simulink model "vehicles"  (Simulink 6.5)
settings: Solver=ode45  StartTime=0.0  StopTime=50  FixedStep=.1  RelTol=1e-3
PreLoadFcn:
  | vehicledata; % load in workspace variables
  | h=frontend; % bring up GUI
  | movegui(h,'northwest') % move gui to top right
PostLoadFcn:
  | rt=sfroot; chart=rt.find('-isa', 'Stateflow.Chart', '-and', 'Name','uav_modes'); chart.view;
undefined symbols (not defined in the file or in its folder): Cd0, Clmax, Clmin, g, initthis, k, magnitude, mat2cell, num_ac, num_instincts, obstacles, omega_chi, omega_gamma, omega_v, rho, S, sigma_a, sigma_o, sigma_t1, sigma_t2, targets, Tmax, W
libraries: dspmtrx3 x38, dspindex x5, dspstat3 x4, vrlib x2
(part 2 of 2)

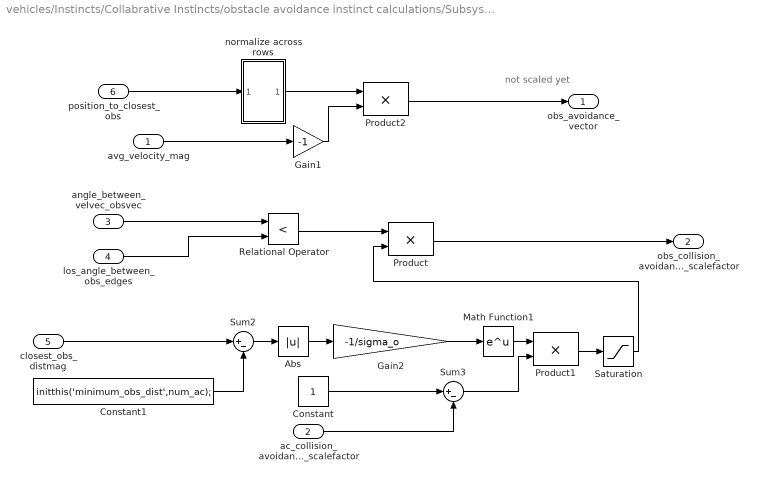
== system vehicles/Instincts/Collabrative Instincts/obstacle avoidance instinct calculations/Subsystem ==
  note: not scaled yet
  avg_velocity_mag : Inport
  ac_collision_avoidance_scalefactor : Inport  Port=2
  angle_between_velvec_obsvec : Inport  Port=3
  los_angle_between_obs_edges : Inport  Port=4
  closest_obs_distmag : Inport  Port=5
  position_to_closest_obs : Inport  Port=6
  Abs : Abs  SaturateOnIntegerOverflow=on  SampleTime=-1
  Constant : Constant  Value=1  OutDataType=sfix(16)  ConRadixGroup=Use specified scaling  OutScaling=2^0  SampleTime=inf  FramePeriod=inf
  Constant1 : Constant  Value=initthis('minimum_obs_dist',num_ac);  OutDataType=sfix(16)  ConRadixGroup=Use specified scaling  OutScaling=2^0  SampleTime=inf  FramePeriod=inf
  Gain1 : Gain  Gain=-1  SaturateOnIntegerOverflow=on
  Gain2 : Gain  Gain=-1/sigma_o  SaturateOnIntegerOverflow=on
  Math Function1 : Math  SaturateOnIntegerOverflow=on
  Product : Product  SaturateOnIntegerOverflow=on  InputSameDT=on
  Product1 : Product  SaturateOnIntegerOverflow=on  InputSameDT=on
  Product2 : Product  SaturateOnIntegerOverflow=on  InputSameDT=on
  Relational Operator : RelationalOperator  Operator=<  InputSameDT=on
  Saturation : Saturate  UpperLimit=1  LowerLimit=0
  Sum2 : Sum  Inputs=|+-  SaturateOnIntegerOverflow=on  InputSameDT=on
  Sum3 : Sum  Inputs=|+-  SaturateOnIntegerOverflow=on  InputSameDT=on
  normalize across rows : Subsystem
  obs_avoidance_vector : Outport
  obs_collision_avoidance_scalefactor : Outport  Port=2
  wires:
  angle_between_velvec_obsvec/1 -> Relational Operator/1
  los_angle_between_obs_edges/1 -> Relational Operator/2
  Relational Operator/1 -> Product/1
  closest_obs_distmag/1 -> Sum2/1
  Constant1/1 -> Sum2/2
  Sum2/1 -> Abs/1
  Gain2/1 -> Math Function1/1
  Abs/1 -> Gain2/1
  Constant/1 -> Sum3/1
  ac_collision_avoidance_scalefactor/1 -> Sum3/2
  Math Function1/1 -> Product1/1
  Sum3/1 -> Product1/2
  Product1/1 -> Saturation/1
  Saturation/1 -> Product/2
  Product/1 -> obs_collision_avoidance_scalefactor/1
  position_to_closest_obs/1 -> normalize across rows/1(In1)
  normalize across rows/1(Out1) -> Product2/1
  avg_velocity_mag/1 -> Gain1/1
  Gain1/1 -> Product2/2
  Product2/1 -> obs_avoidance_vector/1

== system vehicles/Instincts/Collabrative Instincts/target aquisition instinct calculations/desired heading and velocity capture ==
  In1 : Inport
  Abs : Abs  SaturateOnIntegerOverflow=on  SampleTime=-1
  Constant1 : Constant  Value=initthis('desired_vel',num_ac);  OutDataType=sfix(16)  ConRadixGroup=Use specified scaling  OutScaling=2^0  SampleTime=inf  FramePeriod=inf
  Constant3 : Constant  Value=1  OutDataType=sfix(16)  ConRadixGroup=Use specified scaling  OutScaling=2^0  SampleTime=inf  FramePeriod=inf
  Gain1 : Gain  Gain=-1  SaturateOnIntegerOverflow=on
  Gain2 : Gain  Gain=1/sigma_t1  SaturateOnIntegerOverflow=on
  Math Function1 : Math  Operator=sqrt  SaturateOnIntegerOverflow=on
  Math Function2 : Math  Operator=square  SaturateOnIntegerOverflow=on
  Math Function4 : Math  Operator=square  SaturateOnIntegerOverflow=on
  Math Function5 : Math  SaturateOnIntegerOverflow=on
  Matrix Sum : dspmtrx3/Matrix Sum  DialogController=dspDDGCreate  DialogControllerArgs=DataTag15  Dim=Rows  roundingMode=Floor  overflowMode=off
  Sum1 : Sum  Inputs=|+-  SaturateOnIntegerOverflow=on  InputSameDT=on
  Sum2 : Sum  Inputs=|+-  SaturateOnIntegerOverflow=on  InputSameDT=on
  "[x_dot y_dot h_dot]" : Subsystem
  velocity vectors of each AC : Concatenate  NumInputs=3  Mode=Horizontal matrix concatenation
  desired_velvec1 : Outport
  tgt_aquire_scalefactor1 : Outport  Port=2
  wires:
  "[x_dot y_dot h_dot]"/3(h_dot) -> velocity vectors of each AC/3
  "[x_dot y_dot h_dot]"/2(y_dot) -> velocity vectors of each AC/2
  "[x_dot y_dot h_dot]"/1(x_dot) -> velocity vectors of each AC/1
  velocity vectors of each AC/1 -> Sum1/2
  Sum1/1 -> Math Function2/1
  Math Function2/1 -> Matrix Sum/1
  Math Function1/1 -> [vel_error_mag]
  Matrix Sum/1 -> Math Function1/1
  [vel_error_mag] -> Gain2/1
  Gain2/1 -> Math Function4/1
  Math Function4/1 -> Gain1/1
  Math Function5/1 -> Sum2/1
  Constant3/1 -> Sum2/2
  Sum2/1 -> Abs/1
  In1/1 -> "[x_dot y_dot h_dot]"/1(States)
  Abs/1 -> tgt_aquire_scalefactor1/1
  Gain1/1 -> Math Function5/1
  Constant1/1 -> Sum1/1, desired_velvec1/1

== system vehicles/Instincts/Collabrative Instincts/target aquisition instinct calculations/target capture ==
  In1 : Inport
  In2 : Inport  Port=2
  tgt_aquire_on : Inport  Port=3
  If : If
  If Action Subsystem : Subsystem  TreatAsAtomicUnit=on
  If Action Subsystem1 : Subsystem  TreatAsAtomicUnit=on
  Merge : Merge
  Merge1 : Merge
  Transpose : dspmtrx3/Transpose  SystemSampleTime=-1  Hermitian=off  overflowFlag=on
  tgt_aquire_scalefactor2 : Outport
  desired_velvec2 : Outport  Port=2
  wires:
  tgt_aquire_on/1 -> If/1
  If/1 -> If Action Subsystem/Action
  If/2 -> If Action Subsystem1/Action
  If Action Subsystem/1(tgt_aquire_scalefactor2) -> Merge/1
  If Action Subsystem1/1(tgt_aquire_scalefactor2) -> Merge/2
  If Action Subsystem1/2(desired_velvec2) -> Merge1/2
  If Action Subsystem/2(desired_velvec2) -> Merge1/1
  Merge/1 -> Transpose/1
  In1/1 -> If Action Subsystem/1(States)
  In2/1 -> If Action Subsystem/2(avg_velocity_mag)
  Transpose/1 -> tgt_aquire_scalefactor2/1
  Merge1/1 -> desired_velvec2/1

== system vehicles/Vehicle/EOM/[Velocity_dot gamma_dot chi_dot]/Subsystem ==
  Velocity : Inport
  loadfactor : Inport  Port=2
  Gain1 : Gain  Gain=.5*rho*S*Cd0  SaturateOnIntegerOverflow=on
  Gain2 : Gain  Gain=2*k*W^2/(rho*S)  SaturateOnIntegerOverflow=on
  Math Function : Math  Operator=square  SaturateOnIntegerOverflow=on
  Math Function1 : Math  Operator=square  SaturateOnIntegerOverflow=on
  Product : Product  Inputs=/*  SaturateOnIntegerOverflow=on  InputSameDT=on
  Sum : Sum  Inputs=|++  SaturateOnIntegerOverflow=on  InputSameDT=on
  Drag : Outport
  wires:
  Velocity/1 -> Math Function/1
  Math Function/1 -> Gain1/1, Product/1
  loadfactor/1 -> Math Function1/1
  Math Function1/1 -> Product/2
  Product/1 -> Gain2/1
  Gain2/1 -> Sum/2
  Gain1/1 -> Sum/1
  Sum/1 -> Drag/1

== system vehicles/Instincts/Collabrative Instincts/AC avoidance instinct calculations/Distance between AC Calculator1/For Iterator Subsystem ==
  num_ac : Inport
  positions : Inport  Port=2
  position : Inport  Port=3
  initial row : Inport  Port=4
  row : Inport  Port=5
  Assignment : Assignment  InputType=Matrix  IndexIsStartValue=off  ElementSrc=External  Elements=1  RowSrc=Internal  Rows=1  ColumnSrc=External  Columns=1  OutputDimensions=[1 1]
  Constant : Constant  Value=1e099  OutDataType=sfix(16)  ConRadixGroup=Use specified scaling  OutScaling=2^0  SampleTime=inf  FramePeriod=inf
  For Iterator : ForIterator  IterationSource=external  IterationVariableDataType=double
  Math Function : Math  Operator=magnitude^2  SaturateOnIntegerOverflow=on
  Math Function1 : Math  Operator=sqrt  SaturateOnIntegerOverflow=on
  Matrix Sum : dspmtrx3/Matrix Sum  DialogController=dspDDGCreate  DialogControllerArgs=DataTag1  Dim=Rows  roundingMode=Floor  overflowMode=off
  Relational Operator : RelationalOperator  Operator===  InputSameDT=on
  Selector : Selector  InputType=Matrix  ElementSrc=Internal  Elements=[1 3]  RowSrc=External  Rows=1  ColumnSrc=Internal  Columns=-1  InputPortWidth=3  IndexIsStartValue=off
  Sum : Sum  Inputs=|-+  SaturateOnIntegerOverflow=on  InputSameDT=on
  Switch1 : Switch  Threshold=.5  SaturateOnIntegerOverflow=on  InputSameDT=on
  row for one aircraft : Outport
  wires:
  num_ac/1 -> For Iterator/1
  For Iterator/1 -> Selector/2, Relational Operator/1, Assignment/3
  positions/1 -> Selector/1
  position/1 -> Sum/1
  Selector/1 -> Sum/2
  Sum/1 -> Math Function/1
  Math Function/1 -> Matrix Sum/1
  Matrix Sum/1 -> Math Function1/1
  Relational Operator/1 -> Switch1/2
  Switch1/1 -> Assignment/2
  Math Function1/1 -> Switch1/3
  Constant/1 -> Switch1/1
  row/1 -> Relational Operator/2
  initial row/1 -> Assignment/1
  Assignment/1 -> row for one aircraft/1

== system vehicles/Instincts/Collabrative Instincts/obstacle avoidance instinct calculations/Angle calulator/[x_dot y_dot h_dot] ==
  States : Inport
  Product : Product  Inputs=3  SaturateOnIntegerOverflow=on  InputSameDT=on
  Product1 : Product  SaturateOnIntegerOverflow=on  InputSameDT=on
  Product2 : Product  Inputs=3  SaturateOnIntegerOverflow=on  InputSameDT=on
  "V, gamma, chi" : BusSelector  OutputSignals=Velocity,gamma,chi
  cos_chi : Trigonometry  Operator=cos
  cos_gamma : Trigonometry  Operator=cos
  sin_chi : Trigonometry
  sin_gamma : Trigonometry
  x_dot : Outport
  y_dot : Outport  Port=2
  h_dot : Outport  Port=3
  wires:
  "V, gamma, chi"/1 -> Product2/1, Product/1, Product1/1  "<Velocity>"
  "V, gamma, chi"/2 -> sin_gamma/1, cos_gamma/1  "<gamma>"
  "V, gamma, chi"/3 -> sin_chi/1, cos_chi/1  "<chi>"
  cos_gamma/1 -> Product2/2, Product/2
  cos_chi/1 -> Product2/3
  sin_chi/1 -> Product/3
  sin_gamma/1 -> Product1/2
  States/1 -> "V, gamma, chi"/1
  Product2/1 -> x_dot/1  "x_dot"
  Product/1 -> y_dot/1  "y_dot"
  Product1/1 -> h_dot/1  "h_dot"

== system vehicles/Instincts/Collabrative Instincts/obstacle avoidance instinct calculations/Angle calulator/normalize across rows ==
  In1 : Inport
  Math Function : Math  Operator=square  SaturateOnIntegerOverflow=on
  Math Function1 : Math  Operator=sqrt  SaturateOnIntegerOverflow=on
  Math Function2 : Math  Operator=reciprocal  SaturateOnIntegerOverflow=on
  Matrix Scaling : dspmtrx3/Matrix Scaling  DialogController=dspDDGCreate  DialogControllerArgs=DataTag7  mode=Scale rows (D*A)  D_Source=Input port  D_VectFromMask=[0.5 0.25]  roundingMode=Floor  overflowMode=off
  Matrix Sum : dspmtrx3/Matrix Sum  DialogController=dspDDGCreate  DialogControllerArgs=DataTag8  Dim=Rows  roundingMode=Floor  overflowMode=off
  Out1 : Outport
  wires:
  In1/1 -> Matrix Scaling/1, Math Function/1
  Math Function/1 -> Matrix Sum/1
  Matrix Sum/1 -> Math Function1/1
  Math Function1/1 -> Math Function2/1
  Math Function2/1 -> Matrix Scaling/2
  Matrix Scaling/1 -> Out1/1

== system vehicles/Instincts/Collabrative Instincts/obstacle avoidance instinct calculations/Angle calulator/normalize across rows1 ==
  In1 : Inport
  Math Function : Math  Operator=square  SaturateOnIntegerOverflow=on
  Math Function1 : Math  Operator=sqrt  SaturateOnIntegerOverflow=on
  Math Function2 : Math  Operator=reciprocal  SaturateOnIntegerOverflow=on
  Matrix Scaling : dspmtrx3/Matrix Scaling  DialogController=dspDDGCreate  DialogControllerArgs=DataTag9  mode=Scale rows (D*A)  D_Source=Input port  D_VectFromMask=[0.5 0.25]  roundingMode=Floor  overflowMode=off
  Matrix Sum : dspmtrx3/Matrix Sum  DialogController=dspDDGCreate  DialogControllerArgs=DataTag10  Dim=Rows  roundingMode=Floor  overflowMode=off
  Out1 : Outport
  wires:
  In1/1 -> Matrix Scaling/1, Math Function/1
  Math Function/1 -> Matrix Sum/1
  Matrix Sum/1 -> Math Function1/1
  Math Function1/1 -> Math Function2/1
  Math Function2/1 -> Matrix Scaling/2
  Matrix Scaling/1 -> Out1/1

== system vehicles/Instincts/Collabrative Instincts/obstacle avoidance instinct calculations/Distance from obstacles Calculator/For Iterator Subsystem ==
  note: filling in columns at a time.
      | ie distance to each obstacle from
      | a given aircraft.
      | [num_obs, num_ac]
  position of obs : Inport
  num_obs : Inport  Port=2
  position of ac : Inport  Port=3
  initial column : Inport  Port=4
  Assignment : Assignment  InputType=Vector  IndexIsStartValue=off  ElementSrc=External  Elements=1  RowSrc=External  Rows=1  ColumnSrc=External  Columns=1  OutputDimensions=[1 1]
  For Iterator : ForIterator  IterationSource=external  IterationVariableDataType=double
  Math Function : Math  Operator=magnitude^2  SaturateOnIntegerOverflow=on
  Math Function1 : Math  Operator=sqrt  SaturateOnIntegerOverflow=on
  Matrix Sum : dspmtrx3/Matrix Sum  DialogController=dspDDGCreate  DialogControllerArgs=DataTag11  Dim=Rows  roundingMode=Floor  overflowMode=off
  Selector : Selector  InputType=Matrix  ElementSrc=Internal  Elements=[1 3]  RowSrc=External  Rows=1  ColumnSrc=Internal  Columns=-1  InputPortWidth=3  IndexIsStartValue=off
  Sum : Sum  Inputs=|-+  SaturateOnIntegerOverflow=on  InputSameDT=on
  row for one obstacle : Outport
  wires:
  num_obs/1 -> For Iterator/1
  For Iterator/1 -> Selector/2, Assignment/3
  position of obs/1 -> Selector/1
  position of ac/1 -> Sum/1
  Selector/1 -> Sum/2
  Sum/1 -> Math Function/1
  Math Function/1 -> Matrix Sum/1
  Matrix Sum/1 -> Math Function1/1
  Math Function1/1 -> Assignment/2
  initial column/1 -> Assignment/1
  Assignment/1 -> row for one obstacle/1

== system vehicles/Instincts/Collabrative Instincts/obstacle avoidance instinct calculations/Subsystem/normalize across rows ==
  In1 : Inport
  Math Function : Math  Operator=square  SaturateOnIntegerOverflow=on
  Math Function1 : Math  Operator=sqrt  SaturateOnIntegerOverflow=on
  Math Function2 : Math  Operator=reciprocal  SaturateOnIntegerOverflow=on
  Matrix Scaling : dspmtrx3/Matrix Scaling  DialogController=dspDDGCreate  DialogControllerArgs=DataTag13  mode=Scale rows (D*A)  D_Source=Input port  D_VectFromMask=[0.5 0.25]  roundingMode=Floor  overflowMode=off
  Matrix Sum : dspmtrx3/Matrix Sum  DialogController=dspDDGCreate  DialogControllerArgs=DataTag14  Dim=Rows  roundingMode=Floor  overflowMode=off
  Out1 : Outport
  wires:
  In1/1 -> Matrix Scaling/1, Math Function/1
  Math Function/1 -> Matrix Sum/1
  Matrix Sum/1 -> Math Function1/1
  Math Function1/1 -> Math Function2/1
  Math Function2/1 -> Matrix Scaling/2
  Matrix Scaling/1 -> Out1/1

== system vehicles/Instincts/Collabrative Instincts/target aquisition instinct calculations/desired heading and velocity capture/[x_dot y_dot h_dot] ==
  States : Inport
  Product : Product  Inputs=3  SaturateOnIntegerOverflow=on  InputSameDT=on
  Product1 : Product  SaturateOnIntegerOverflow=on  InputSameDT=on
  Product2 : Product  Inputs=3  SaturateOnIntegerOverflow=on  InputSameDT=on
  "V, gamma, chi" : BusSelector  OutputSignals=Velocity,gamma,chi
  cos_chi : Trigonometry  Operator=cos
  cos_gamma : Trigonometry  Operator=cos
  sin_chi : Trigonometry
  sin_gamma : Trigonometry
  x_dot : Outport
  y_dot : Outport  Port=2
  h_dot : Outport  Port=3
  wires:
  "V, gamma, chi"/1 -> Product2/1, Product/1, Product1/1  "<Velocity>"
  "V, gamma, chi"/2 -> sin_gamma/1, cos_gamma/1  "<gamma>"
  "V, gamma, chi"/3 -> sin_chi/1, cos_chi/1  "<chi>"
  cos_gamma/1 -> Product2/2, Product/2
  cos_chi/1 -> Product2/3
  sin_chi/1 -> Product/3
  sin_gamma/1 -> Product1/2
  States/1 -> "V, gamma, chi"/1
  Product2/1 -> x_dot/1  "x_dot"
  Product/1 -> y_dot/1  "y_dot"
  Product1/1 -> h_dot/1  "h_dot"

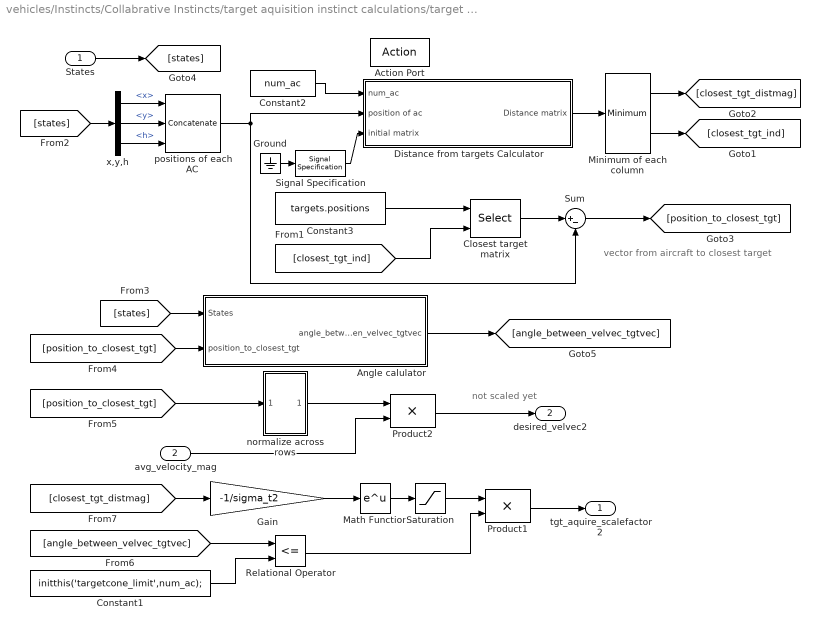
== system vehicles/Instincts/Collabrative Instincts/target aquisition instinct calculations/target capture/If Action Subsystem ==
  note: vector from aircraft to closest target
  note: not scaled yet
  States : Inport
  avg_velocity_mag : Inport  Port=2
  Action Port : ActionPort  ActionType=then
  Angle calulator : Subsystem
  Closest target matrix : Selector  InputType=Matrix  ElementSrc=Internal  Elements=[1 3]  RowSrc=External  Rows=1  ColumnSrc=Internal  Columns=-1  InputPortWidth=3  IndexIsStartValue=off
  Constant1 : Constant  Value=initthis('targetcone_limit',num_ac);  OutDataType=sfix(16)  ConRadixGroup=Use specified scaling  OutScaling=2^0  SampleTime=inf  FramePeriod=inf
  Constant2 : Constant  Value=num_ac  OutDataType=sfix(16)  ConRadixGroup=Use specified scaling  OutScaling=2^0  SampleTime=inf  FramePeriod=inf
  Constant3 : Constant  Value=targets.positions  OutDataType=sfix(16)  ConRadixGroup=Use specified scaling  OutScaling=2^0  SampleTime=inf  FramePeriod=inf
  Distance from targets Calculator : Subsystem  TreatAsAtomicUnit=on
  Gain : Gain  Gain=-1/sigma_t2  SaturateOnIntegerOverflow=on
  Ground : Ground
  Math Function : Math  SaturateOnIntegerOverflow=on
  Minimum of each column : dspstat3/Minimum  DialogController=dspfixptddg.MinMax  DialogControllerArgs=DataTag21  fcn=Value and Index  reset=None  indexBase=One  operateOver=Each column  colComp=on  operation=minimum  roundingMode=Floor  overflowMode=off
  Product1 : Product  SaturateOnIntegerOverflow=on  InputSameDT=on
  Product2 : Product  SaturateOnIntegerOverflow=on  InputSameDT=on
  Relational Operator : RelationalOperator  Operator=<=  InputSameDT=on
  Saturation : Saturate  UpperLimit=1  LowerLimit=0
  Signal Specification : SignalSpecification  Dimensions=[size(targets.positions,1),num_ac]
  Sum : Sum  Inputs=|+-  SaturateOnIntegerOverflow=on  InputSameDT=on
  normalize across rows : Subsystem
  positions of each AC : Concatenate  NumInputs=3  Mode=Horizontal matrix concatenation
  x,y,h : BusSelector  OutputSignals=x,y,h
  tgt_aquire_scalefactor2 : Outport
  desired_velvec2 : Outport  Port=2
  wires:
  Minimum of each column/1 -> [closest_tgt_distmag]
  Sum/1 -> [position_to_closest_tgt]
  Minimum of each column/2 -> [closest_tgt_ind]
  Distance from targets Calculator/1(Distance matrix) -> Minimum of each column/1
  positions of each AC/1 -> Sum/2, Distance from targets Calculator/2(position of ac)
  x,y,h/3 -> positions of each AC/3  "<h>"
  x,y,h/2 -> positions of each AC/2  "<y>"
  x,y,h/1 -> positions of each AC/1  "<x>"
  [closest_tgt_ind] -> Closest target matrix/2
  Constant3/1 -> Closest target matrix/1
  Closest target matrix/1 -> Sum/1
  States/1 -> [states]
  [states] -> x,y,h/1
  [states] -> Angle calulator/1(States)
  [position_to_closest_tgt] -> Angle calulator/2(position_to_closest_tgt)
  Angle calulator/1(angle_between_velvec_tgtvec) -> [angle_between_velvec_tgtvec]
  [position_to_closest_tgt] -> normalize across rows/1(In1)
  normalize across rows/1(Out1) -> Product2/1
  avg_velocity_mag/1 -> Product2/2
  Product2/1 -> desired_velvec2/1
  [angle_between_velvec_tgtvec] -> Relational Operator/1
  Constant1/1 -> Relational Operator/2
  Relational Operator/1 -> Product1/2
  Math Function/1 -> Saturation/1
  [closest_tgt_distmag] -> Gain/1
  Gain/1 -> Math Function/1
  Saturation/1 -> Product1/1
  Product1/1 -> tgt_aquire_scalefactor2/1
  Ground/1 -> Signal Specification/1
  Constant2/1 -> Distance from targets Calculator/1(num_ac)
  Signal Specification/1 -> Distance from targets Calculator/3(initial matrix)

== system vehicles/Instincts/Collabrative Instincts/target aquisition instinct calculations/target capture/If Action Subsystem1 ==
  Action Port : ActionPort  ActionType=else
  Ground : Ground
  Ground1 : Ground
  Signal Specification : SignalSpecification  Dimensions=[num_ac]
  Signal Specification1 : SignalSpecification  Dimensions=[num_ac,3]
  tgt_aquire_scalefactor2 : Outport
  desired_velvec2 : Outport  Port=2
  wires:
  Ground/1 -> Signal Specification/1
  Signal Specification/1 -> tgt_aquire_scalefactor2/1
  Signal Specification1/1 -> desired_velvec2/1
  Ground1/1 -> Signal Specification1/1

== system vehicles/Instincts/Collabrative Instincts/target aquisition instinct calculations/target capture/If Action Subsystem/Angle calulator ==
  States : Inport
  position_to_closest_tgt : Inport  Port=2
  Extract Diagonal : dspmtrx3/Extract Diagonal
  Matrix Multiply : Product  Multiplication=Matrix(*)
  Transpose1 : dspmtrx3/Transpose  SystemSampleTime=-1  Hermitian=off  overflowFlag=on
  Trigonometric Function : Trigonometry  Operator=acos
  "[x_dot y_dot h_dot]" : Subsystem
  normalize across rows : Subsystem
  normalize across rows1 : Subsystem
  velocity vectors of each AC : Concatenate  NumInputs=3  Mode=Horizontal matrix concatenation
  angle_between_velvec_tgtvec : Outport
  wires:
  "[x_dot y_dot h_dot]"/3(h_dot) -> velocity vectors of each AC/3
  "[x_dot y_dot h_dot]"/2(y_dot) -> velocity vectors of each AC/2
  "[x_dot y_dot h_dot]"/1(x_dot) -> velocity vectors of each AC/1
  velocity vectors of each AC/1 -> normalize across rows/1(In1)
  normalize across rows/1(Out1) -> Matrix Multiply/1
  normalize across rows1/1(Out1) -> Transpose1/1
  Transpose1/1 -> Matrix Multiply/2
  Matrix Multiply/1 -> Extract Diagonal/1
  Extract Diagonal/1 -> Trigonometric Function/1
  States/1 -> "[x_dot y_dot h_dot]"/1(States)
  Trigonometric Function/1 -> angle_between_velvec_tgtvec/1
  position_to_closest_tgt/1 -> normalize across rows1/1(In1)

== system vehicles/Instincts/Collabrative Instincts/target aquisition instinct calculations/target capture/If Action Subsystem/Distance from targets Calculator ==
  num_ac : Inport
  position of ac : Inport  Port=2
  initial matrix : Inport  Port=3
  Assignment : Assignment  InputType=Matrix  IndexIsStartValue=off  ElementSrc=External  Elements=1  RowSrc=External  Rows=1  ColumnSrc=External  Columns=1  OutputDimensions=[1 1]
  Constant : Constant  Value=[1:size(targets.positions,1)]  OutDataType=sfix(16)  ConRadixGroup=Use specified scaling  OutScaling=2^0  SampleTime=inf  FramePeriod=inf
  Constant1 : Constant  Value=targets.positions  OutDataType=sfix(16)  ConRadixGroup=Use specified scaling  OutScaling=2^0  SampleTime=inf  FramePeriod=inf
  Constant2 : Constant  Value=size(targets.positions,1)  OutDataType=sfix(16)  ConRadixGroup=Use specified scaling  OutScaling=2^0  SampleTime=inf  FramePeriod=inf
  For Iterator : ForIterator  IterationSource=external  IterationVariableDataType=double
  For Iterator Subsystem : Subsystem  TreatAsAtomicUnit=on
  Ground : Ground
  Selector : Selector  InputType=Matrix  ElementSrc=Internal  Elements=[1 3]  RowSrc=External  Rows=1  ColumnSrc=Internal  Columns=-1  InputPortWidth=3  IndexIsStartValue=off
  Signal Specification : SignalSpecification  Dimensions=[size(targets.positions,1),1]
  Distance matrix : Outport
  wires:
  num_ac/1 -> For Iterator/1
  For Iterator/1 -> Selector/2, Assignment/4
  position of ac/1 -> Selector/1
  Selector/1 -> For Iterator Subsystem/3(position of ac)
  For Iterator Subsystem/1(column for one target) -> Assignment/2
  Ground/1 -> Signal Specification/1
  Signal Specification/1 -> For Iterator Subsystem/4(initial column)
  initial matrix/1 -> Assignment/1
  Assignment/1 -> Distance matrix/1
  Constant1/1 -> For Iterator Subsystem/1(position of tgt)
  Constant/1 -> Assignment/3
  Constant2/1 -> For Iterator Subsystem/2(num_tgt)

== system vehicles/Instincts/Collabrative Instincts/target aquisition instinct calculations/target capture/If Action Subsystem/normalize across rows ==
  In1 : Inport
  Math Function : Math  Operator=square  SaturateOnIntegerOverflow=on
  Math Function1 : Math  Operator=sqrt  SaturateOnIntegerOverflow=on
  Math Function2 : Math  Operator=reciprocal  SaturateOnIntegerOverflow=on
  Matrix Scaling : dspmtrx3/Matrix Scaling  DialogController=dspDDGCreate  DialogControllerArgs=DataTag22  mode=Scale rows (D*A)  D_Source=Input port  D_VectFromMask=[0.5 0.25]  roundingMode=Floor  overflowMode=off
  Matrix Sum : dspmtrx3/Matrix Sum  DialogController=dspDDGCreate  DialogControllerArgs=DataTag23  Dim=Rows  roundingMode=Floor  overflowMode=off
  Out1 : Outport
  wires:
  In1/1 -> Matrix Scaling/1, Math Function/1
  Math Function/1 -> Matrix Sum/1
  Matrix Sum/1 -> Math Function1/1
  Math Function1/1 -> Math Function2/1
  Math Function2/1 -> Matrix Scaling/2
  Matrix Scaling/1 -> Out1/1

== system vehicles/Instincts/Collabrative Instincts/target aquisition instinct calculations/target capture/If Action Subsystem/Angle calulator/[x_dot y_dot h_dot] ==
  States : Inport
  Product : Product  Inputs=3  SaturateOnIntegerOverflow=on  InputSameDT=on
  Product1 : Product  SaturateOnIntegerOverflow=on  InputSameDT=on
  Product2 : Product  Inputs=3  SaturateOnIntegerOverflow=on  InputSameDT=on
  "V, gamma, chi" : BusSelector  OutputSignals=Velocity,gamma,chi
  cos_chi : Trigonometry  Operator=cos
  cos_gamma : Trigonometry  Operator=cos
  sin_chi : Trigonometry
  sin_gamma : Trigonometry
  x_dot : Outport
  y_dot : Outport  Port=2
  h_dot : Outport  Port=3
  wires:
  "V, gamma, chi"/1 -> Product2/1, Product/1, Product1/1  "<Velocity>"
  "V, gamma, chi"/2 -> sin_gamma/1, cos_gamma/1  "<gamma>"
  "V, gamma, chi"/3 -> sin_chi/1, cos_chi/1  "<chi>"
  cos_gamma/1 -> Product2/2, Product/2
  cos_chi/1 -> Product2/3
  sin_chi/1 -> Product/3
  sin_gamma/1 -> Product1/2
  States/1 -> "V, gamma, chi"/1
  Product2/1 -> x_dot/1  "x_dot"
  Product/1 -> y_dot/1  "y_dot"
  Product1/1 -> h_dot/1  "h_dot"

== system vehicles/Instincts/Collabrative Instincts/target aquisition instinct calculations/target capture/If Action Subsystem/Angle calulator/normalize across rows ==
  In1 : Inport
  Math Function : Math  Operator=square  SaturateOnIntegerOverflow=on
  Math Function1 : Math  Operator=sqrt  SaturateOnIntegerOverflow=on
  Math Function2 : Math  Operator=reciprocal  SaturateOnIntegerOverflow=on
  Matrix Scaling : dspmtrx3/Matrix Scaling  DialogController=dspDDGCreate  DialogControllerArgs=DataTag16  mode=Scale rows (D*A)  D_Source=Input port  D_VectFromMask=[0.5 0.25]  roundingMode=Floor  overflowMode=off
  Matrix Sum : dspmtrx3/Matrix Sum  DialogController=dspDDGCreate  DialogControllerArgs=DataTag17  Dim=Rows  roundingMode=Floor  overflowMode=off
  Out1 : Outport
  wires:
  In1/1 -> Matrix Scaling/1, Math Function/1
  Math Function/1 -> Matrix Sum/1
  Matrix Sum/1 -> Math Function1/1
  Math Function1/1 -> Math Function2/1
  Math Function2/1 -> Matrix Scaling/2
  Matrix Scaling/1 -> Out1/1

== system vehicles/Instincts/Collabrative Instincts/target aquisition instinct calculations/target capture/If Action Subsystem/Angle calulator/normalize across rows1 ==
  In1 : Inport
  Math Function : Math  Operator=square  SaturateOnIntegerOverflow=on
  Math Function1 : Math  Operator=sqrt  SaturateOnIntegerOverflow=on
  Math Function2 : Math  Operator=reciprocal  SaturateOnIntegerOverflow=on
  Matrix Scaling : dspmtrx3/Matrix Scaling  DialogController=dspDDGCreate  DialogControllerArgs=DataTag18  mode=Scale rows (D*A)  D_Source=Input port  D_VectFromMask=[0.5 0.25]  roundingMode=Floor  overflowMode=off
  Matrix Sum : dspmtrx3/Matrix Sum  DialogController=dspDDGCreate  DialogControllerArgs=DataTag19  Dim=Rows  roundingMode=Floor  overflowMode=off
  Out1 : Outport
  wires:
  In1/1 -> Matrix Scaling/1, Math Function/1
  Math Function/1 -> Matrix Sum/1
  Matrix Sum/1 -> Math Function1/1
  Math Function1/1 -> Math Function2/1
  Math Function2/1 -> Matrix Scaling/2
  Matrix Scaling/1 -> Out1/1

== system vehicles/Instincts/Collabrative Instincts/target aquisition instinct calculations/target capture/If Action Subsystem/Distance from targets Calculator/For Iterator Subsystem ==
  note: filling in columns at a time.
      | ie distance to each target from
      | a given aircraft.
      | [num_tgt, num_ac]
  position of tgt : Inport
  num_tgt : Inport  Port=2
  position of ac : Inport  Port=3
  initial column : Inport  Port=4
  Assignment : Assignment  InputType=Vector  IndexIsStartValue=off  ElementSrc=External  Elements=1  RowSrc=External  Rows=1  ColumnSrc=External  Columns=1  OutputDimensions=[1 1]
  For Iterator : ForIterator  IterationSource=external  IterationVariableDataType=double
  Math Function : Math  Operator=magnitude^2  SaturateOnIntegerOverflow=on
  Math Function1 : Math  Operator=sqrt  SaturateOnIntegerOverflow=on
  Matrix Sum : dspmtrx3/Matrix Sum  DialogController=dspDDGCreate  DialogControllerArgs=DataTag20  Dim=Rows  roundingMode=Floor  overflowMode=off
  Selector : Selector  InputType=Matrix  ElementSrc=Internal  Elements=[1 3]  RowSrc=External  Rows=1  ColumnSrc=Internal  Columns=-1  InputPortWidth=3  IndexIsStartValue=off
  Sum : Sum  Inputs=|-+  SaturateOnIntegerOverflow=on  InputSameDT=on
  column for one target : Outport
  wires:
  num_tgt/1 -> For Iterator/1
  For Iterator/1 -> Selector/2, Assignment/3
  position of tgt/1 -> Selector/1
  position of ac/1 -> Sum/1
  Selector/1 -> Sum/2
  Sum/1 -> Math Function/1
  Math Function/1 -> Matrix Sum/1
  Matrix Sum/1 -> Math Function1/1
  Math Function1/1 -> Assignment/2
  initial column/1 -> Assignment/1
  Assignment/1 -> column for one target/1

== stateflow chart Mode Display/uav_modes ==
  state uav1 [parallel]
    settings: executionOrder=1
    state ac_avoid
      en:mode_count[1][1]++;
    state obs_avoid
      en:mode_count[1][2]++;
    state tgt_aquire
      en:mode_count[1][3]++;
    state form_keep
      en:mode_count[1][4]++;
    uav1 -> uav1.ac_avoid [order 1] : aa
    uav1 -> uav1.obs_avoid [order 2] : oa
    uav1 -> uav1.form_keep [order 4] : fk
    uav1 -> uav1.tgt_aquire [order 3] : ta
    (default) -> uav1.ac_avoid
  state uav2 [parallel]
    settings: executionOrder=2
    state ac_avoid
      en:mode_count[2][1]++;
    state obs_avoid
      en:mode_count[2][2]++;
    state tgt_aquire
      en:mode_count[2][3]++;
    state form_keep
      en:mode_count[2][4]++;
    uav2 -> uav2.ac_avoid [order 1] : aa
    uav2 -> uav2.obs_avoid [order 2] : oa
    uav2 -> uav2.form_keep [order 4] : fk
    uav2 -> uav2.tgt_aquire [order 3] : ta
    (default) -> uav2.ac_avoid
  state uav3 [parallel]
    settings: executionOrder=3
    state ac_avoid
      en:mode_count[3][1]++;
    state obs_avoid
      en:mode_count[3][2]++;
    state tgt_aquire
      en:mode_count[3][3]++;
    state form_keep
      en:mode_count[3][4]++;
    uav3 -> uav3.ac_avoid [order 1] : aa
    uav3 -> uav3.obs_avoid [order 2] : oa
    uav3 -> uav3.form_keep [order 4] : fk
    uav3 -> uav3.tgt_aquire [order 3] : ta
    (default) -> uav3.ac_avoid
  state uav4 [parallel]
    settings: executionOrder=4
    state ac_avoid
      en:mode_count[4][1]++;
    state obs_avoid
      en:mode_count[4][2]++;
    state tgt_aquire
      en:mode_count[4][3]++;
    state form_keep
      en:mode_count[4][4]++;
    uav4 -> uav4.ac_avoid [order 1] : aa
    uav4 -> uav4.obs_avoid [order 2] : oa
    uav4 -> uav4.form_keep [order 4] : fk
    uav4 -> uav4.tgt_aquire [order 3] : ta
    (default) -> uav4.ac_avoid
  state uav5 [parallel]
    settings: executionOrder=5
    state ac_avoid
      en:mode_count[5][1]++;
    state obs_avoid
      en:mode_count[5][2]++;
    state tgt_aquire
      en:mode_count[5][3]++;
    state form_keep
      en:mode_count[5][4]++;
    uav5 -> uav5.ac_avoid [order 1] : aa
    uav5 -> uav5.obs_avoid [order 2] : oa
    uav5 -> uav5.form_keep [order 4] : fk
    uav5 -> uav5.tgt_aquire [order 3] : ta
    (default) -> uav5.ac_avoid
  state parse_events [parallel]
    on e1: uav1.aa;
    on e2: uav1.oa;
    on e3: uav1.ta;
    on e4: uav1.fk;
    on e5: uav2.aa;
    on e6: uav2.oa;
    on e7: uav2.ta;
    on e8: uav2.fk;
    on e9: uav3.aa;
    on e10: uav3.oa;
    on e11: uav3.ta;
    on e12: uav3.fk;
    on e13: uav4.aa;
    on e14: uav4.oa;
    on e15: uav4.ta;
    on e16: uav4.fk;
    on e17: uav5.aa;
    on e18: uav5.oa;
    on e19: uav5.ta;
    on e20: uav5.fk;
    settings: executionOrder=6
  data: mode_count local double size=[5 4]
  events: aa local EITHER_EDGE_EVENT; fk local EITHER_EDGE_EVENT; oa local EITHER_EDGE_EVENT; ta local EITHER_EDGE_EVENT; aa local EITHER_EDGE_EVENT; fk local EITHER_EDGE_EVENT; oa local EITHER_EDGE_EVENT; ta local EITHER_EDGE_EVENT; aa local EITHER_EDGE_EVENT; fk local EITHER_EDGE_EVENT; oa local EITHER_EDGE_EVENT; ta local EITHER_EDGE_EVENT; aa local EITHER_EDGE_EVENT; fk local EITHER_EDGE_EVENT; oa local EITHER_EDGE_EVENT; ta local EITHER_EDGE_EVENT; aa local EITHER_EDGE_EVENT; fk local EITHER_EDGE_EVENT; oa local EITHER_EDGE_EVENT; ta local EITHER_EDGE_EVENT; e1 input RISING_EDGE_EVENT; e2 input RISING_EDGE_EVENT; e3 input RISING_EDGE_EVENT; e4 input RISING_EDGE_EVENT; e5 input RISING_EDGE_EVENT; e6 input RISING_EDGE_EVENT; e7 input RISING_EDGE_EVENT; e8 input RISING_EDGE_EVENT; e9 input RISING_EDGE_EVENT; e10 input RISING_EDGE_EVENT; e11 input RISING_EDGE_EVENT; e12 input RISING_EDGE_EVENT; e13 input RISING_EDGE_EVENT; e14 input RISING_EDGE_EVENT; e15 input RISING_EDGE_EVENT; e16 input RISING_EDGE_EVENT; e17 input RISING_EDGE_EVENT; e18 input RISING_EDGE_EVENT; e19 input RISING_EDGE_EVENT; e20 input RISING_EDGE_EVENT
